simulink model "imageUDPNode_th"  (R2018b)
settings: Solver=FixedStepDiscrete  StartTime=0.0  StopTime=inf  FixedStep=0.025  RelTol=1e-3  EnableMultiTasking=on
undefined symbols (not defined in the file): ipaddr, PTP
libraries: ptplib x5, slrtlib x4, xpcutilitieslib x2, xpcrtudplib x2
settings Model: SimulationMode=external  Creator=The MathWorks, Inc.  LastModifiedBy=MAE-NCSUCORE
settings SolverCC: ConcurrentTasks=on  AutoInsertRateTranBlk=on  DecoupledContinuousIntegration=on  MinimalZcImpactIntegration=on
settings DataIOCC: SaveFormat=StructureWithTime
settings OptimizationCC: BlockReduction=off  OptimizeBlockIOStorage=off  BufferReuse=off  GlobalBufferReuse=off  ExpressionFolding=off  LocalBlockOutputs=off  OptimizeDataStoreBuffers=off  BusAssignmentInplaceUpdate=off
settings DebuggingCC: LibraryContextMissingDiagnostic=none
settings HardwareCC: ProdBitPerPointer=32  ProdBitPerSizeT=32  ProdBitPerPtrDiffT=32  ProdLargestAtomicFloat=None  ProdWordSize=32  ProdLongLongMode=on  ProdHWDeviceType=Generic->32-bit x86 compatible
settings SFSimCC: SimUseLocalCustomCode=off
settings RTWCC: SystemTargetFile=slrt.tlc  TemplateMakefile=slrt_default_tmf  Description=Simulink Real-Time  RTWVerbose=off  RTWUseLocalCustomCode=off  CodeExecutionProfiling=on  RTWCompilerOptimization=on
settings SimulinkRealTimeCC: SupportVariableSizeSignals=on  PreserveStateflowLocalDataDimensions=off  RL32LogTETModifier=off  RL32LogBufSizeModifier=1000000  RL32ObjectName=tg2  xPCisDefaultEnv=off  xPCTargetPCEnvName=Machine3  xPCConcurrentTasks=on

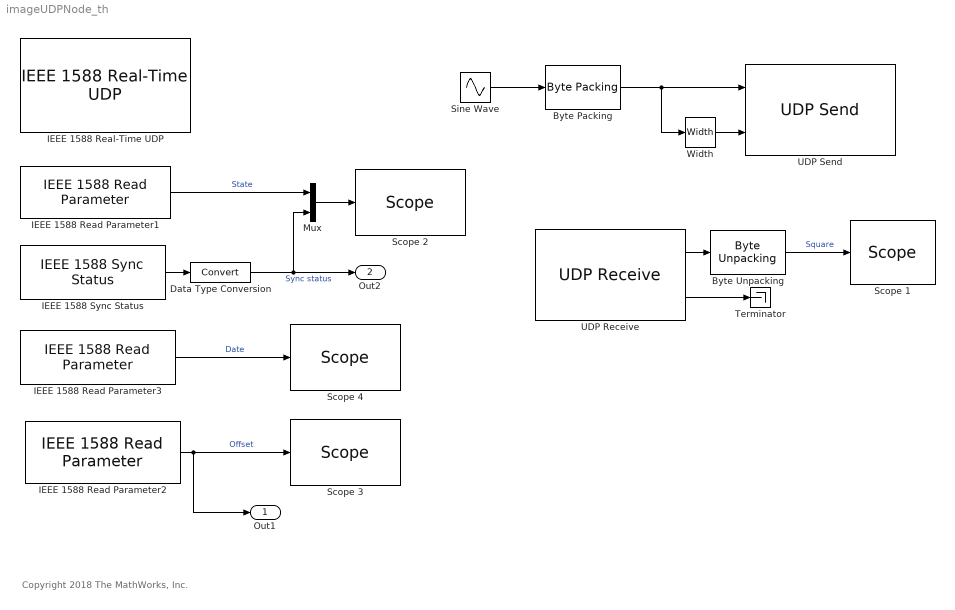
== system imageUDPNode_th ==
  note: Copyright 2018 The MathWorks, Inc.
  "Byte Packing " : xpcutilitieslib/Byte Packing   MaskPackedDataType=uint8  MaskUnpackedDataTypes={'double'}  MaskAlignment=1
  "Byte Unpacking " : xpcutilitieslib/Byte Unpacking   MaskUnpackedDataTypes={'double'}  MaskUnpackedDataSizes={[1]}  MaskAlignment=1
      settings: SourceProductName=Simulink Real-Time  SourceProductBaseCode=XP
  Data Type Conversion : DataTypeConversion
  IEEE 1588 Read Parameter1 : ptplib/IEEE 1588 Read Parameter  Priority=1  ID=1  param=Protocol state  sample_time=0.025  enable_read_precision=off
      settings: SourceProductName=Simulink Real-Time  SourceProductBaseCode=XP
  IEEE 1588 Read Parameter2 : ptplib/IEEE 1588 Read Parameter  Priority=1  ID=1  param=Offset from Master  sample_time=0.025  enable_read_precision=off
      settings: SourceProductName=Simulink Real-Time  SourceProductBaseCode=XP
  IEEE 1588 Read Parameter3 : ptplib/IEEE 1588 Read Parameter  Priority=1  ID=1  param=PTP time (time-of-day)  sample_time=0.025  enable_read_precision=off
      settings: SourceProductName=Simulink Real-Time  SourceProductBaseCode=XP
  IEEE 1588 Sync Status : ptplib/IEEE 1588 Sync Status  Priority=1  ID=1  offset_threshold=10e-6  sample_time=0.025
      settings: SourceProductName=Simulink Real-Time  SourceProductBaseCode=XP
  IEEE 1588 Real-Time UDP : ptplib/IEEE 1588 Real-Time UDP  Priority=0  ID=1  PciBus=4  PciSlot=0  PciFunction=0  time_inc=4000000  sample_time=0.025  IpSource=Specify  IpAddress=30.30.30.1  SubnetMask=255.255.255.0  Gateway=0.0.0.0  Receive1=30.30.30.30  dest_ip_select=Standard PTP multicast (224.0.1.129, 224.0.0.107)  custom_dest_ip_addr=30.30.30.30  MulticastList=[ipaddr('224.0.1.129'), ipaddr('224.0.0.107')]  Multicast={macaddr('01:00:5E:00:01:81'), macaddr('01:00:5E:00:00:6B')}  time_source=Ethernet board  timescale=PTP (1970-01-01)  epoch=[1970 01 01 00]  delay_measure=Request-response  slave_only=off  enable_advanced_config=on  domain_num=0  utc_offset=35  priority1=128  clock_class=248  clock_accuracy=hex2dec('FE')  priority2=128  announce_interval=2  sync_interval=0.1  min_pdelay_req_interval=0.1  announce_receipt_timeout=3
      settings: SourceProductName=Simulink Real-Time  SourceProductBaseCode=XP
  Mux : Mux  Inputs=2
  Scope 1 : slrtlib/Displays and Logging/Scope   scopeno=4  scopetype=Target  autostart=on  viewmode=Graphical rolling  formatstr='%15.6f'  grid=on  ylimits=[0,0]  nosamples=250  noprepostsamples=0  interleave=1  triggermode=FreeRun  triggersignal=1  trigsignalfromport=off  triggerlevel=0.0  triggerslope=Either  triggerscope=1  triggersample=0  filename=data.dat  mode=Lazy  writesize=512  autorestart=off  dynamicfilemode=off  maxwritefilesize=512*1024^2
  Scope 2 : slrtlib/Displays and Logging/Scope   scopeno=1  scopetype=Target  autostart=on  viewmode=Numerical  formatstr='%15.6f'  grid=on  ylimits=[0,0]  nosamples=3  noprepostsamples=0  interleave=1  triggermode=FreeRun  triggersignal=1  trigsignalfromport=off  triggerlevel=0.0  triggerslope=Either  triggerscope=1  triggersample=0  filename=data.dat  mode=Lazy  writesize=512  autorestart=off  dynamicfilemode=off  maxwritefilesize=512*1024^2
  Scope 3 : slrtlib/Displays and Logging/Scope   scopeno=3  scopetype=Target  autostart=on  viewmode=Graphical rolling  formatstr='%15.6f'  grid=on  ylimits=[0,0]  nosamples=250  noprepostsamples=0  interleave=1  triggermode=FreeRun  triggersignal=1  trigsignalfromport=off  triggerlevel=0.0  triggerslope=Either  triggerscope=1  triggersample=0  filename=data.dat  mode=Lazy  writesize=512  autorestart=off  dynamicfilemode=off  maxwritefilesize=512*1024^2
  Scope 4 : slrtlib/Displays and Logging/Scope   scopeno=2  scopetype=Target  autostart=on  viewmode=Numerical  formatstr="'Year:            %-4.0f, Month:           %-4.0f, Day of week:     %-4.0f, Day:             %-4.0f, Hour:            %-4.0f, Minute:          %-4.0f, Second:          %-4.0f, Millisecond:     %-4.0f'"  grid=on  ylimits=[0,0]  nosamples=3  noprepostsamples=0  interleave=1  triggermode=FreeRun  triggersignal=1  trigsignalfromport=off  triggerlevel=0.0  triggerslope=Either  triggerscope=1  triggersample=0  filename=data.dat  mode=Lazy  writesize=512  autorestart=off  dynamicfilemode=off  maxwritefilesize=512*1024^2
  Sine Wave : Sin  Amplitude=10  Frequency=10  SampleTime=0.025
  Terminator : Terminator
  UDP Receive : xpcrtudplib/UDP Receive  ipAddressVal=30.30.30.1  localPort=8000  rcvWidth=8  rcvFmAny=off  fmAddress=30.30.30.30  rcvMulticast=off  multicastAddress={}  maxUDPQueue=8  sampleTime=0.025
      settings: SourceProductName=Simulink Real-Time
  UDP Send : xpcrtudplib/UDP Send  ipAddressVal=30.30.30.1  localPort=-1  toAddress=30.30.30.30  toPort=8001  sampleTime=0.025
      settings: SourceProductName=Simulink Real-Time  SourceProductBaseCode=XP
  Width : Width
  Out1 : Outport
  Out2 : Outport  Port=2
  wires:
  IEEE 1588 Read Parameter1/1 -> Mux/1  "State"
  IEEE 1588 Read Parameter3/1 -> Scope 4/1  "Date"
  "Byte Packing "/1 -> Width/1, UDP Send/1
  Sine Wave/1 -> "Byte Packing "/1
  Width/1 -> UDP Send/2
  UDP Receive/1 -> "Byte Unpacking "/1
  UDP Receive/2 -> Terminator/1
  "Byte Unpacking "/1 -> Scope 1/1  "Square"
  IEEE 1588 Read Parameter2/1 -> Out1/1, Scope 3/1  "Offset"
  Mux/1 -> Scope 2/1
  IEEE 1588 Sync Status/1 -> Data Type Conversion/1
  Data Type Conversion/1 -> Out2/1, Mux/2  "Sync status"
